simulink model "dc_motor_starter_design_v3"  (R2025a)
settings: Solver=VariableStepAuto  StartTime=0.0  StopTime=7  RelTol=1e-3
libraries: spsDiodeLib x8, spsMosfetLib x4, spsCurrentMeasurementLib x3, spsDCVoltageSourceLib x2, simulink x2, spsSeriesRLCBranchLib x2, spsACVoltageSourceLib x1, spsDCMachineLib x1, spsGroundLib x1, eePwmGenerator x1, spsVoltageMeasurementLib x1, spspowerguiLib x1
settings Model: Creator=Lenovo  LastModifiedBy=Lenovo

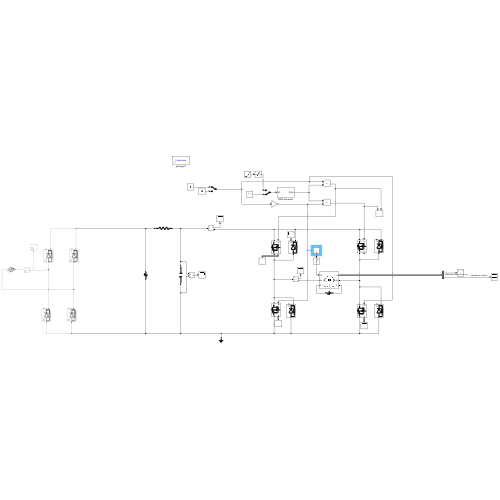
[thumbnail: Simulink's stored preview of the top-level diagram]
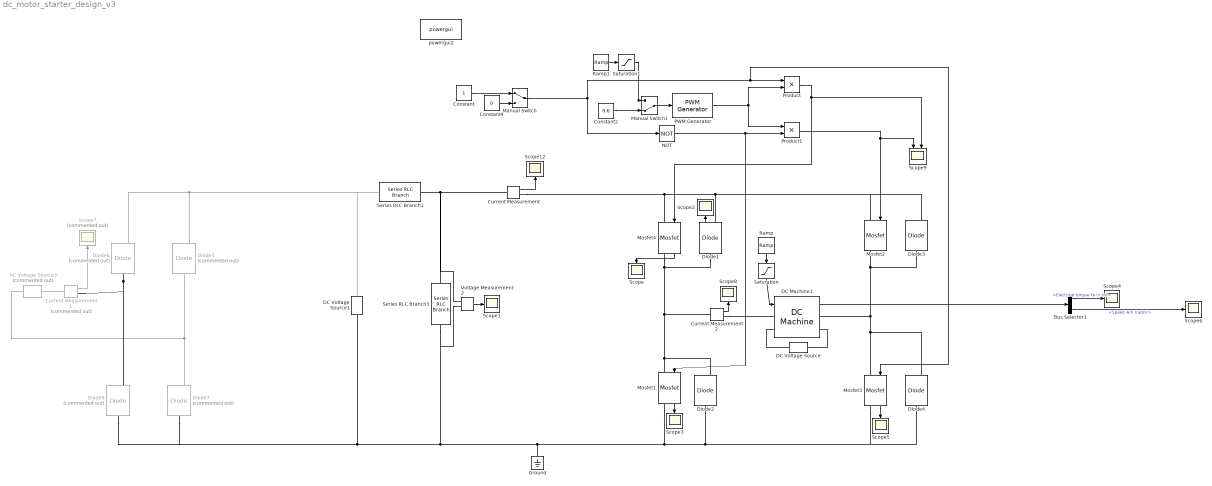
== system dc_motor_starter_design_v3 ==
  AC Voltage Source3 : spsACVoltageSourceLib/AC Voltage Source  Commented=on  Amplitude=205  Phase=0  Frequency=50  SampleTime=0  Measurements=None  BusType=swing  Pref=10e3  Qref=0  Qmin=-inf  Qmax=+inf
  Bus Selector1 : BusSelector  OutputSignals=Electrical torque Te (n m),Speed wm (rad/s)
  Constant : Constant
  Constant2 : Constant  Value=0.6
  Constant4 : Constant  Value=0
  Current Measurement : spsCurrentMeasurementLib/Current Measurement  PhasorSimulation=off  OutputType=Complex  PSBequivalent=0
  Current Measurement1 : spsCurrentMeasurementLib/Current Measurement  Commented=on  PhasorSimulation=off  OutputType=Complex  PSBequivalent=0
  Current Measurement2 : spsCurrentMeasurementLib/Current Measurement  PhasorSimulation=off  OutputType=Complex  PSBequivalent=0
  DC Machine1 : spsDCMachineLib/DC Machine  PresetModel=No  MechanicalLoad=Torque TL  FieldType=Wound  ShowDetailedParameters=on  MeasurementBus=off  RLa="[ 0.8  0.0125]"  RLf="[ 210  23]"  Laf=1.8  MachineConstant=Torque constant (N.m/A)  Ke=1.8  Kt=1.8  J=1  Bm=0  Tf=0  w0=1  Ifinit=1.04761904761905  TsPowergui=0  TsBlock=-1
  DC Voltage Source : spsDCVoltageSourceLib/DC Voltage Source  Amplitude=220  Measurements=None
  DC Voltage Source1 : spsDCVoltageSourceLib/DC Voltage Source  Amplitude=200  Measurements=None
  Diode{1..4} (4 alike) : spsDiodeLib/Diode  Ron=0.036  Lon=0  Vf=1.1  IC=0  UseSnubber=0  Rs=500  Cs=250e-9  Measurements=on
  Diode{5..8} (4 alike) : spsDiodeLib/Diode  Commented=on  Ron=0.036  Lon=0  Vf=1.1  IC=0  UseSnubber=0  Rs=500  Cs=250e-9  Measurements=on
  Ground : spsGroundLib/Ground  LConnTagsString=a
  Manual Switch : ManualSwitch
  Manual Switch1 : ManualSwitch  CurrentSetting=0
  Mosfet{1..4} (4 alike) : spsMosfetLib/Mosfet  Ron=0.078  Lon=0  Rd=0.01  Vfd=0.7  IC=0  Rs=1e5  Cs=inf  Measurements=on
  NOT : Logic  Operator=NOT  IconShape=distinctive  AllPortsSameDT=off  OutDataTypeStr=boolean
  PWM Generator : eePwmGenerator/PWM Generator  CarrCount=Up  Tper=1/20e3  Tdelay=0  Ts=5e-6
  Product : Product
  Product1 : Product
  Ramp : simulink/Sources/Ramp  slope=20  start=5  InitialOutput=0
  Ramp1 : simulink/Sources/Ramp  slope=0.2  start=0  InitialOutput=0
  Saturation : Saturate  UpperLimit=10  LowerLimit=0
  Saturation1 : Saturate  UpperLimit=0.8  LowerLimit=0
  Scope{,1..6,8,12} (9 alike) : Scope
      Scope settings: ActiveDisplayYMinimum=-25.17424958813524  ActiveDisplayYMaximum=226.88170800102853  DataLoggingVariableName=ScopeData2
      Scope1 settings: ActiveDisplayYMinimum=197.20667546347846  ActiveDisplayYMaximum=205.7174886404658
      Scope12 settings: ActiveDisplayYMinimum=-4.3267096598487811  ActiveDisplayYMaximum=9.5444979024542747  DataLoggingVariableName=ScopeData11
      Scope2 settings: ActiveDisplayYMinimum=-226.88562627237616  ActiveDisplayYMaximum=25.20951403026401  DataLoggingVariableName=ScopeData3
      Scope3 settings: DataLoggingVariableName=ScopeData4
      Scope4 settings: ActiveDisplayYMinimum=-32.104324896778238  ActiveDisplayYMaximum=157.67027544286611
      Scope5 settings: ActiveDisplayYMinimum=-1.20703950016334  ActiveDisplayYMaximum=7.0075960496809362  DataLoggingVariableName=ScopeData6
      Scope6 settings: ActiveDisplayYMinimum=-7.1846961495374888  ActiveDisplayYMaximum=74.662265345837412  DataLoggingVariableName=ScopeData5
      Scope8 settings: ActiveDisplayYMinimum=4.773629027337261  ActiveDisplayYMaximum=5.5941548045396914  DataLoggingVariableName=ScopeData8
  Scope7 : Scope  Commented=on
      settings: ActiveDisplayYMinimum=-568.37134406736811  ActiveDisplayYMaximum=546.71556577016588  DataLoggingVariableName=ScopeData7
  Scope9 : Scope  NumInputPorts=2
      settings: ActiveDisplayYMinimum=-0.33686308177258728  ActiveDisplayYMaximum=1.1825197307274133  DataLoggingVariableName=ScopeData9
  Series RLC Branch1 : spsSeriesRLCBranchLib/Series RLC Branch  LConnTagsString=__new0  RConnTagsString=__new0  BranchType=R  Resistance=0.001  Inductance=1e-3  SetiL0=off  InitialCurrent=0  Capacitance=15000e-6  Setx0=off  InitialVoltage=0  Measurements=None
  Series RLC Branch3 : spsSeriesRLCBranchLib/Series RLC Branch  LConnTagsString=__new0  RConnTagsString=__new0  BranchType=C  Resistance=1  Inductance=1e-3  SetiL0=off  InitialCurrent=0  Capacitance=1500e-6  Setx0=off  InitialVoltage=0  Measurements=None
  Voltage Measurement2 : spsVoltageMeasurementLib/Voltage Measurement  PhasorSimulation=off  OutputType=Complex  PSBequivalent=0
  powergui2 : spspowerguiLib/powergui  Priority=1  SimulationMode=Continuous  SampleTime=50e-6  frequency=60  Iterations=50  frequencyindice=0  Pbase=100e6  ErrMax=1e-4  UnitsV=kV  UnitsW=MW  buscounter=0  FunctionMessages=off  echomessages=off  EnableUseOfTLC=off  CurrentSourceSwitches=off  DisableSnubberDevices=off  DisableRonSwitches=off  DisableVfSwitches=off  DisplayEquations=off  AutomaticDiscreteSolvers=off  SolverType=Tustin/Backward Euler (TBE)  Interpol=off  ExternalGateDelay=off  methode=off  Ts=100  x0status=blocks  SPID=on  SwTol=0  HookPort=off  NonlinearTolerance=1e-4  nMaxIteration=100  ContinueOnMaxIteration=off  RestoreLinks=warning  ResistiveCurrentMeasurement=off  Frange=[0:2:500]  Ylog=off  Xlog=on  ShowGrid=off  save=off  variable=ZData  structure=0  ZoomFFT=off  StartTime=0.0  cycles=1  DisplayStyle=1  fundamental=60  FreqAxis=off  MaxFrequency=1000  frequencyindicesteady=1  RmsSteady=1  display=off
  wires:
  Current Measurement1/1 -> Scope7/1
  Voltage Measurement2/1 -> Scope1/1
  Current Measurement/1 -> Scope12/1
  Constant/1 -> Manual Switch/1
  Constant4/1 -> Manual Switch/2
  PWM Generator/1 -> Product1/1, Product/2
  Manual Switch/1 -> NOT/1, Product/1, Mosfet3/1
  NOT/1 -> Product1/2, Mosfet1/1
  Bus Selector1/2 -> Scope6/1  "<Speed wm (rad/s)>"
  Bus Selector1/1 -> Scope4/1  "<Electrical torque Te (n m)>"
  Ramp/1 -> Saturation/1
  DC Machine1/1 -> Bus Selector1/1
  Saturation/1 -> DC Machine1/1
  Ramp1/1 -> Saturation1/1
  Constant2/1 -> Manual Switch1/2
  Saturation1/1 -> Manual Switch1/1
  Manual Switch1/1 -> PWM Generator/1
  Product1/1 -> Scope9/1, Mosfet2/1
  Product/1 -> Scope9/2, Mosfet4/1
  Mosfet4/1 -> Scope/1
  Diode1/1 -> Scope2/1
  Mosfet1/1 -> Scope3/1
  Mosfet3/1 -> Scope5/1
  Current Measurement2/1 -> Scope8/1
  connections:
  AC Voltage Source3/LConn1 -- Diode7/RConn1 -- Diode5/LConn1
  Diode6/LConn1 -- Diode8/RConn1 -- Current Measurement1/RConn1
  Mosfet4/RConn1 -- Diode1/LConn1 -- Current Measurement2/LConn1 -- Diode2/RConn1 -- Mosfet1/LConn1
  AC Voltage Source3/RConn1 -- Current Measurement1/LConn1
  Diode1/RConn1 -- Diode3/RConn1 -- Mosfet2/LConn1 -- Mosfet4/LConn1 -- Current Measurement/RConn1
  Diode8/LConn1 -- Diode7/LConn1 -- DC Voltage Source1/LConn1 -- Mosfet1/RConn1 -- Mosfet3/RConn1 -- Diode4/LConn1 -- Diode2/LConn1 -- Ground/LConn1 -- Voltage Measurement2/LConn2 -- Series RLC Branch3/RConn1
  DC Voltage Source/LConn1 -- DC Machine1/RConn2
  DC Voltage Source/RConn1 -- DC Machine1/LConn2
  Diode5/RConn1 -- Series RLC Branch1/LConn1 -- DC Voltage Source1/RConn1 -- Diode6/RConn1
  Current Measurement2/RConn1 -- DC Machine1/LConn1
  Mosfet3/LConn1 -- Diode4/RConn1 -- DC Machine1/RConn1 -- Diode3/LConn1 -- Mosfet2/RConn1
  Current Measurement/LConn1 -- Series RLC Branch1/RConn1 -- Voltage Measurement2/LConn1 -- Series RLC Branch3/LConn1
